simulink model "psbnetsim2"  (Simulink 6.0)
settings: Solver=ode23s  SolverMode=SingleTasking  StartTime=0.0  StopTime=0.06  RelTol=1e-3  AbsTol=1e-6
libraries: powerlib2 x8, powerlib_extras x1
settings Model: Creator=patrice  LastModifiedBy=batserve  ExtModeTrigMode=oneshot  ExtModeArmWhenConnect=off  ExtModeAutoUpdateStatusClock=off
settings DataIOCC: LimitDataPoints=off  SignalLoggingName=sigsOut
settings OptimizationCC: BooleanDataType=off
settings DebuggingCC: SolverPrmCheckMsg=none
settings HardwareCC: TargetUnknown=on
settings RTWCC: TemplateMakefile=grt_unix.tmf

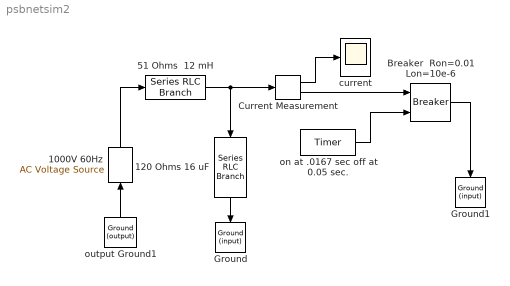
== system psbnetsim2 ==
  1000V 60Hz : powerlib2/Electrical Sources/AC Voltage Source  Tag=PoWeRsYsTeMbLoCk  Orientation=up  A=1000  P=0  F=60  stime=0  mesure=None  PSBOutputType=1
  "120 Ohms 16 uF " : powerlib2/Elements/Series RLC Branch  Tag=PoWeRsYsTeMbLoCk  Orientation=down  a=120  b=0  c=16e-06  mesure=None  PSBOutputType=1
  51 Ohms  12 mH : powerlib2/Elements/Series RLC Branch  Tag=PoWeRsYsTeMbLoCk  a=51  b=12e-03  c=inf  mesure=None  PSBOutputType=1
  Breaker  Ron=0.01 Lon=10e-6 : powerlib2/Elements/Breaker  Tag=PoWeRsYsTeMbLoCk  a=0.01  c=0  rs=inf  cs=0  times="[ 4/60  5/60 ]"  Ts=0  comext=on  mesure=None  PSBOutputType=1
  Current Measurement : powerlib2/Measurements/Current Measurement  Tag=PoWeRsYsTeMmEaSuReMeNt  PhasorSimulation=off  OutputType=Magnitude  PSBOutputType=01  PSBequivalent=0
  Ground : powerlib2/Connectors/Ground (input)  Tag=PoWeRsYsTeMbLoCk  Orientation=down
  Ground1 : powerlib2/Connectors/Ground (input)  Tag=PoWeRsYsTeMbLoCk  Orientation=down
  current : Scope
      settings: TickLabels=on  TimeRange=0.06  YMin=-20  YMax=20  DataFormat=Array
  on at .0167 sec off at 0.05 sec. : powerlib_extras/Control  Blocks/Timer  t=[0 1/60 3/60]  e=[0 1 0 ]
  output Ground1 : powerlib2/Connectors/Ground (output)  Tag=PoWeRsYsTeMbLoCk  Orientation=up  PSBOutputType=1
  wires:
  51 Ohms  12 mH/1 -> Current Measurement/1, "120 Ohms 16 uF "/1
  "120 Ohms 16 uF "/1 -> Ground/1
  Current Measurement/1 -> current/1
  Breaker  Ron=0.01 Lon=10e-6/1 -> Ground1/1
  Current Measurement/2 -> Breaker  Ron=0.01 Lon=10e-6/1
  1000V 60Hz/1 -> 51 Ohms  12 mH/1
  output Ground1/1 -> 1000V 60Hz/1
  on at .0167 sec off at 0.05 sec./1 -> Breaker  Ron=0.01 Lon=10e-6/2
